simulink model "DraftSimpleEstimatorANDControl"  (R2021b)
settings: Solver=ode1  StartTime=0.0  StopTime=inf  FixedStep=10e-3  RelTol=1e-3
libraries: TcTargetLib x19, slpidlib x1
settings Model: Creator=Mergin  LastModifiedBy=ATLabor
settings OptimizationCC: DefaultParameterBehavior=Inlined  LocalBlockOutputs=off
settings DebuggingCC: UnconnectedInputMsg=none  UnconnectedOutputMsg=none  UnconnectedLineMsg=none
settings ModelReferenceCC: EnableRefExpFcnMdlSchedulingChecks=off
settings RTWCC: Description=TwinCAT GRT Target  SystemTargetFile=TwinCatGrt.tlc  GenCodeOnly=on  TemplateMakefile=tcgrt_msbuild.tmf  TargetLang=C++  DLArmComputeVersion=20.02.1
settings STFCustomTargetCC: TargetLangStandard=C++11 (ISO)  CombineOutputUpdateFcns=on  CodeInterfacePackaging=Reusable function  CPPClassGenCompliant=on  GRTInterface=off  GenerateAllocFcn=on  SystemTargetFile=TwinCatGrt.tlc
settings GRTTargetCC: TargetLangStandard=C++11 (ISO)  ParMdlRefBuildCompliant=off  CompOptLevelCompliant=off  ConcurrentExecutionCompliant=off  MatFileLogging=off  CodeInterfacePackaging=Reusable function  GenerateAllocFcn=on  UseToolchainInfoCompliant=off  ExtModeMexFile=TcExtModeClient

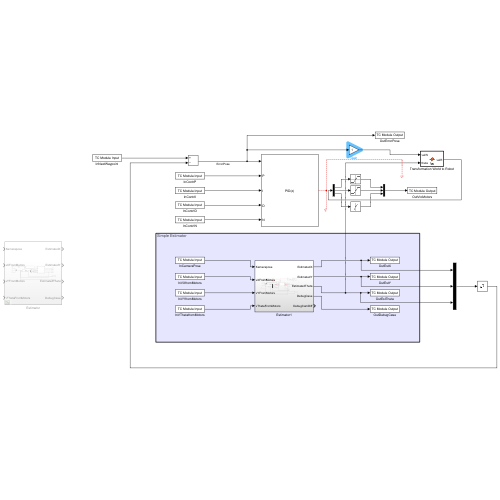
[thumbnail: Simulink's stored preview of the top-level diagram]
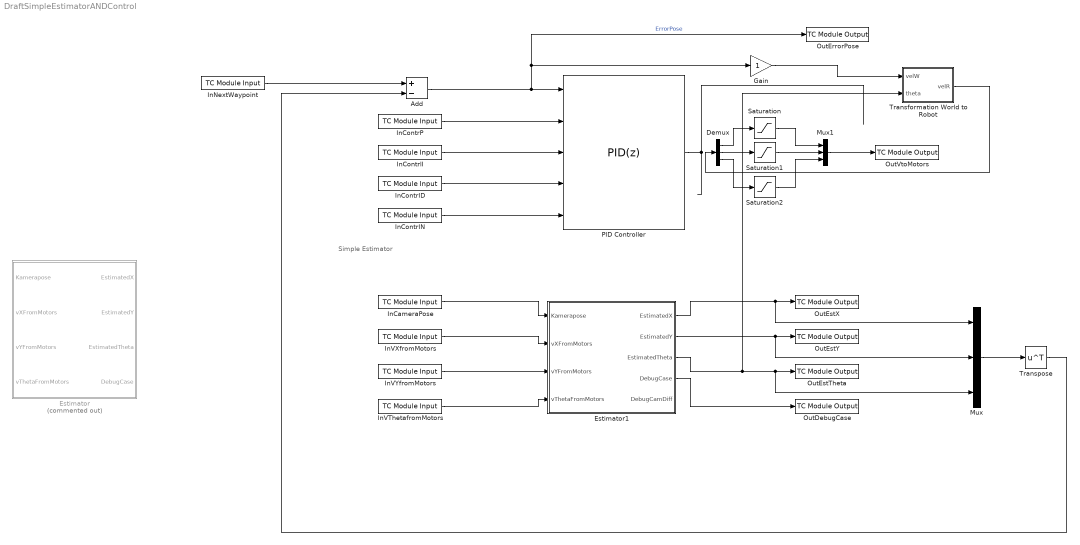
== system DraftSimpleEstimatorANDControl ==
  note: Simple Estimator
  Add : Sum  Inputs=+-
  Demux : Demux  Outputs=3
  Estimator : Subsystem  Commented=on
  Estimator1 : Subsystem
  Gain : Gain
  InCameraPose : TcTargetLib/TC Module Input  PortDataType=double  PortDim=3  Value=[0 0 0]  SampleTime=-1  CodeGenConnectType=DataArea (InputDst)  DataTypeOverride=on
      settings: SourceProductName=Beckhoff TwinCAT Target
  InContrID : TcTargetLib/TC Module Input  PortDataType=double  PortDim=1  Value=0  SampleTime=-1  CodeGenConnectType=DataArea (InputDst)  DataTypeOverride=off
      settings: SourceProductName=Beckhoff TwinCAT Target
  InContrIN : TcTargetLib/TC Module Input  PortDataType=double  PortDim=1  Value=0  SampleTime=-1  CodeGenConnectType=DataArea (InputDst)  DataTypeOverride=off
      settings: SourceProductName=Beckhoff TwinCAT Target
  InContrP : TcTargetLib/TC Module Input  PortDataType=double  PortDim=1  Value=0  SampleTime=-1  CodeGenConnectType=DataArea (InputDst)  DataTypeOverride=off
      settings: SourceProductName=Beckhoff TwinCAT Target
  InContrlI : TcTargetLib/TC Module Input  PortDataType=double  PortDim=1  Value=0  SampleTime=-1  CodeGenConnectType=DataArea (InputDst)  DataTypeOverride=off
      settings: SourceProductName=Beckhoff TwinCAT Target
  InNextWaypoint : TcTargetLib/TC Module Input  PortDataType=double  PortDim=3  Value=[0; 0; 0]  SampleTime=-1  CodeGenConnectType=DataArea (InputDst)  DataTypeOverride=off
      settings: SourceProductName=Beckhoff TwinCAT Target
  InVThetafromMotors : TcTargetLib/TC Module Input  PortDataType=double  PortDim=1  Value=0  SampleTime=-1  CodeGenConnectType=DataArea (InputDst)  DataTypeOverride=off
      settings: SourceProductName=Beckhoff TwinCAT Target
  InVXfromMotors : TcTargetLib/TC Module Input  PortDataType=double  PortDim=1  Value=0  SampleTime=-1  CodeGenConnectType=DataArea (InputDst)  DataTypeOverride=off
      settings: SourceProductName=Beckhoff TwinCAT Target
  InVYfromMotors : TcTargetLib/TC Module Input  PortDataType=double  PortDim=1  Value=0  SampleTime=-1  CodeGenConnectType=DataArea (InputDst)  DataTypeOverride=off
      settings: SourceProductName=Beckhoff TwinCAT Target
  Mux : Mux  Inputs=3
  Mux1 : Mux  Inputs=3
  OutDebugCase : TcTargetLib/TC Module Output  PortDataType=double  PortDim=1  SampleTime=-1  CodeGenConnectType=DataArea (OutputSrc)  DataTypeOverride=off
      settings: SourceProductName=Beckhoff TwinCAT Target
  OutErrorPose : TcTargetLib/TC Module Output  PortDataType=double  PortDim=3  SampleTime=-1  CodeGenConnectType=DataArea (OutputSrc)  DataTypeOverride=off
      settings: SourceProductName=Beckhoff TwinCAT Target
  OutEstTheta : TcTargetLib/TC Module Output  PortDataType=double  PortDim=1  SampleTime=-1  CodeGenConnectType=DataArea (OutputSrc)  DataTypeOverride=off
      settings: SourceProductName=Beckhoff TwinCAT Target
  OutEstX : TcTargetLib/TC Module Output  PortDataType=double  PortDim=1  SampleTime=-1  CodeGenConnectType=DataArea (OutputSrc)  DataTypeOverride=off
      settings: SourceProductName=Beckhoff TwinCAT Target
  OutEstY : TcTargetLib/TC Module Output  PortDataType=double  PortDim=1  SampleTime=-1  CodeGenConnectType=DataArea (OutputSrc)  DataTypeOverride=off
      settings: SourceProductName=Beckhoff TwinCAT Target
  OutVtoMotors : TcTargetLib/TC Module Output  PortDataType=double  PortDim=3  SampleTime=-1  CodeGenConnectType=DataArea (OutputSrc)  DataTypeOverride=off
      settings: SourceProductName=Beckhoff TwinCAT Target
  PID Controller : slpidlib/PID Controller  Controller=PID  Form=Parallel  TimeDomain=Discrete-time  UseExternalTs=off  SampleTime=-1  IntegratorMethod=Forward Euler  FilterMethod=Forward Euler  ControllerParametersSource=external  P=1  I=1  D=0  UseFilter=on  N=100  TunerSelectOption=Transfer Function Based (PID Tuner App)  InitialConditionSource=internal  InitialConditionForIntegrator=0  InitialConditionForFilter=0  DifferentiatorICPrevScaledInput=0  ExternalReset=none  TrackingMode=off  Kt=1  LimitOutput=off  SatLimitsSource=internal  UpperSaturationLimit=inf  LowerSaturationLimit=-inf  LinearizeAsGain=on  AntiWindupMode=none  Kb=1  POutMin=[]  POutMax=[]  IOutMin=[]  IOutMax=[]  DOutMin=[]  DOutMax=[]  NOutMin=[]  NOutMax=[]  SumOutMin=[]  SumOutMax=[]  SaturationOutMin=[]  SaturationOutMax=[]  PParamMin=[]  PParamMax=[]  IParamMin=[]  IParamMax=[]  DParamMin=[]  DParamMax=[]  NParamMin=[]  NParamMax=[]  KbParamMin=[]  KbParamMax=[]  KtParamMin=[]  KtParamMax=[]  KbOutMin=[]  KbOutMax=[]  KtOutMin=[]  KtOutMax=[]  IntegratorOutMin=[]  IntegratorOutMax=[]  FilterOutMin=[]  FilterOutMax=[]  SumI1OutMin=[]  SumI1OutMax=[]  SumI2OutMin=[]  SumI2OutMax=[]  SumI3OutMin=[]  SumI3OutMax=[]  SumI4OutMin=[]  SumI4OutMax=[]  SumDOutMin=[]  SumDOutMax=[]  DifferentiatorOutMin=[]  DifferentiatorOutMax=[]  FilterDiffOutCoefMin=[]  FilterDiffOutCoefMax=[]  ReciprocalOutMin=[]  ReciprocalOutMax=[]  SumDenOutMin=[]  SumDenOutMax=[]  SumNumOutMin=[]  SumNumOutMax=[]  DivideOutMin=[]  DivideOutMax=[]  UdiffTsProdOutMin=[]  UdiffTsProdOutMax=[]  NTsProdOutMin=[]  NTsProdOutMax=[]  UintegralTsProdOutMin=[]  UintegralTsProdOutMax=[]  UngainTsProdOutMin=[]  UngainTsProdOutMax=[]  IntegratorContinuousStateAttributes=''  IntegratorStateMustResolveToSignalObject=off  IntegratorRTWStateStorageClass=Auto  FilterContinuousStateAttributes=''  FilterStateMustResolveToSignalObject=off  FilterRTWStateStorageClass=Auto  ParallelPVariant=ExternalParameters  IdealPVariant=Disabled  IVariant=ExternalParameters  DVariant=ExternalParameters  IntegratorVariant=Discrete  SatVariant=Disabled  AWVariant=Passthrough  PCopyVariant=Disabled  TRVariant=Disabled  FdbkBlocksVariant=Forward  IdealPFdbkVariant=Disabled  SatFdbkVariant=Disabled  DerivativeFilterVariant=ForwardEulerFilter  NVariant=ExternalParameters  NCopyVariant=Disabled  FilterICVariant=InternalICsFilter  IntegratorICVariant=InternalICs  ExternalResetVariant=Disabled  TRSumVariant=Passthrough  SumFdbkVariant=Disabled  SumVariant=Sum_PID  TsampFilterVariant=InternalTs  TsampNgainVariant=Passthrough  TsampIntegralVariant=Passthrough  ExternalSaturationOutDataTypeStr=Inherit: Same as second input
  Saturation : Saturate  UpperLimit=500  LowerLimit=-500
  Saturation1 : Saturate  UpperLimit=500  LowerLimit=-500
  Saturation2 : Saturate  UpperLimit=1  LowerLimit=-1
  Transformation World to Robot : MATLAB Function  TreatAsAtomicUnit=on
  Transpose : Math  Operator=transpose  SaturateOnIntegerOverflow=on
  wires:
  InCameraPose/1 -> Estimator1/1(Kamerapose)
  InVXfromMotors/1 -> Estimator1/2(vXFromMotors)
  InVYfromMotors/1 -> Estimator1/3(vYFromMotors)
  InVThetafromMotors/1 -> Estimator1/4(vThetaFromMotors)
  Estimator1/4(DebugCase) -> OutDebugCase/1
  InContrP/1 -> PID Controller/2
  InContrlI/1 -> PID Controller/3
  InContrID/1 -> PID Controller/4
  InContrIN/1 -> PID Controller/5
  InNextWaypoint/1 -> Add/1
  Add/1 -> Gain/1, OutErrorPose/1, PID Controller/1  "ErrorPose"
  Estimator1/1(EstimatedX) -> OutEstX/1, Mux/1
  Transpose/1 -> Add/2
  Estimator1/2(EstimatedY) -> OutEstY/1, Mux/2
  Mux/1 -> Transpose/1
  Estimator1/3(EstimatedTheta) -> Transformation World to Robot/2(theta), OutEstTheta/1, Mux/3
  PID Controller/1 -> ?
  Demux/1 -> Saturation/1
  Saturation/1 -> Mux1/1
  Demux/2 -> Saturation1/1
  Saturation1/1 -> Mux1/2
  Demux/3 -> Saturation2/1
  Saturation2/1 -> Mux1/3
  Gain/1 -> Transformation World to Robot/1(velW)
  Mux1/1 -> OutVtoMotors/1
  Transformation World to Robot/1(velR) -> Demux/1

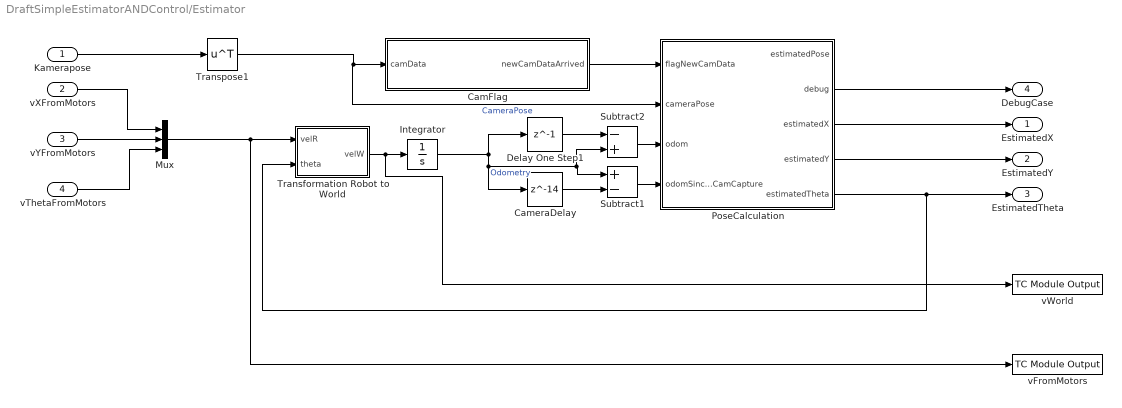
== system DraftSimpleEstimatorANDControl/Estimator ==
  Kamerapose : Inport
  vXFromMotors : Inport  Port=2
  vYFromMotors : Inport  Port=3
  vThetaFromMotors : Inport  Port=4
  CamFlag : MATLAB Function  TreatAsAtomicUnit=on
  CameraDelay : Delay  DelayLength=14
  Delay One Step1 : Delay  DelayLength=1
  Integrator : Integrator
  Mux : Mux  Inputs=3
  PoseCalculation : MATLAB Function  TreatAsAtomicUnit=on
  Subtract1 : Sum  Inputs=+-
  Subtract2 : Sum  Inputs=-+
  Transformation Robot to World : MATLAB Function  TreatAsAtomicUnit=on
  Transpose1 : Math  Operator=transpose  SaturateOnIntegerOverflow=on
  vFromMotors : TcTargetLib/TC Module Output  PortDataType=double  PortDim=3  SampleTime=-1  CodeGenConnectType=DataArea (OutputSrc)  DataTypeOverride=off
      settings: SourceProductName=Beckhoff TwinCAT Target
  vWorld : TcTargetLib/TC Module Output  PortDataType=double  PortDim=3  SampleTime=-1  CodeGenConnectType=DataArea (OutputSrc)  DataTypeOverride=off
      settings: SourceProductName=Beckhoff TwinCAT Target
  EstimatedX : Outport
  EstimatedY : Outport  Port=2
  EstimatedTheta : Outport  Port=3
  DebugCase : Outport  Port=4
  wires:
  vThetaFromMotors/1 -> Mux/3
  Subtract1/1 -> PoseCalculation/4(odomSinceCamCapture)
  CameraDelay/1 -> Subtract1/2
  Transformation Robot to World/1(velW) -> vWorld/1, Integrator/1
  vXFromMotors/1 -> Mux/1
  Transpose1/1 -> CamFlag/1(camData), PoseCalculation/2(cameraPose)  "CameraPose"
  Integrator/1 -> Delay One Step1/1, CameraDelay/1, Subtract2/2, Subtract1/1  "Odometry"
  vYFromMotors/1 -> Mux/2
  CamFlag/1(newCamDataArrived) -> PoseCalculation/1(flagNewCamData)
  Kamerapose/1 -> Transpose1/1
  Delay One Step1/1 -> Subtract2/1
  Subtract2/1 -> PoseCalculation/3(odom)
  PoseCalculation/2(debug) -> DebugCase/1
  Mux/1 -> Transformation Robot to World/1(velR), vFromMotors/1
  PoseCalculation/4(estimatedY) -> EstimatedY/1
  PoseCalculation/3(estimatedX) -> EstimatedX/1
  PoseCalculation/5(estimatedTheta) -> Transformation Robot to World/2(theta), EstimatedTheta/1

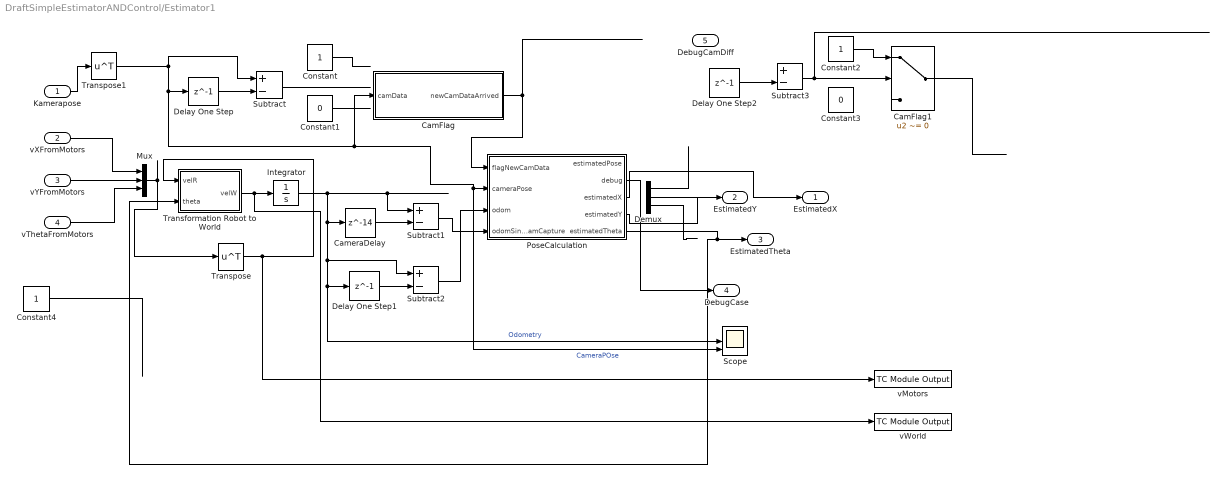
== system DraftSimpleEstimatorANDControl/Estimator1 ==
  Kamerapose : Inport
  vXFromMotors : Inport  Port=2
  vYFromMotors : Inport  Port=3
  vThetaFromMotors : Inport  Port=4
  CamFlag : MATLAB Function  TreatAsAtomicUnit=on
  CamFlag1 : Switch  Criteria=u2 ~= 0
  CameraDelay : Delay  DelayLength=14
  Constant : Constant
  Constant1 : Constant  Value=0
  Constant2 : Constant
  Constant3 : Constant  Value=0
  Constant4 : Constant
  Delay One Step : Delay  DelayLength=1
  Delay One Step1 : Delay  DelayLength=1
  Delay One Step2 : Delay  DelayLength=1
  Demux : Demux  Outputs=3
  Integrator : Integrator
  Mux : Mux  Inputs=3
  PoseCalculation : MATLAB Function  TreatAsAtomicUnit=on
  Scope : Scope  NumInputPorts=3
  Subtract{,1..3} (4 alike) : Sum  Inputs=+-
  Transformation Robot to World : MATLAB Function  TreatAsAtomicUnit=on
  Transpose : Math  Operator=transpose  SaturateOnIntegerOverflow=on
  Transpose1 : Math  Operator=transpose  SaturateOnIntegerOverflow=on
  vMotors : TcTargetLib/TC Module Output  PortDataType=double  PortDim=3  SampleTime=-1  CodeGenConnectType=DataArea (OutputSrc)  DataTypeOverride=off
      settings: SourceProductName=Beckhoff TwinCAT Target
  vWorld : TcTargetLib/TC Module Output  PortDataType=double  PortDim=3  SampleTime=-1  CodeGenConnectType=DataArea (OutputSrc)  DataTypeOverride=off
      settings: SourceProductName=Beckhoff TwinCAT Target
  EstimatedX : Outport
  EstimatedY : Outport  Port=2
  EstimatedTheta : Outport  Port=3
  DebugCase : Outport  Port=4
  DebugCamDiff : Outport  Port=5
  wires:
  Demux/1 -> ?
  Constant/1 -> ?
  Delay One Step/1 -> Subtract/2
  Demux/2 -> ?
  vThetaFromMotors/1 -> Mux/3
  Subtract1/1 -> PoseCalculation/4(odomSinceCamCapture)
  Mux/1 -> Transpose/1
  CameraDelay/1 -> Subtract1/2
  Constant1/1 -> ?
  Transformation Robot to World/1(velW) -> vWorld/1, Integrator/1
  vXFromMotors/1 -> Mux/1
  Transpose1/1 -> Scope/3, PoseCalculation/2(cameraPose), CamFlag/1(camData), Delay One Step/1, Subtract/1  "CameraPOse"
  Integrator/1 -> Subtract1/1, Delay One Step1/1, Scope/2, Subtract2/1, CameraDelay/1  "Odometry"
  vYFromMotors/1 -> Mux/2
  CamFlag/1(newCamDataArrived) -> PoseCalculation/1(flagNewCamData)
  ? -> Scope/1, Demux/1
  Subtract/1 -> ?
  Kamerapose/1 -> Transpose1/1
  Delay One Step1/1 -> Subtract2/2
  Subtract2/1 -> PoseCalculation/3(odom)
  PoseCalculation/2(debug) -> DebugCase/1
  Constant2/1 -> CamFlag1/1
  CamFlag1/1 -> ?
  Subtract3/1 -> CamFlag1/2
  ? -> Subtract3/1  "CameraPOse"
  Delay One Step2/1 -> Subtract3/2
  Transpose/1 -> vMotors/1, Transformation Robot to World/1(velR)
  Demux/3 -> ?
  PoseCalculation/4(estimatedY) -> EstimatedY/1
  PoseCalculation/3(estimatedX) -> EstimatedX/1
  Constant4/1 -> ?
  PoseCalculation/5(estimatedTheta) -> Transformation Robot to World/2(theta), EstimatedTheta/1

== matlab function DraftSimpleEstimatorANDControl/Estimator/PoseCalculation ==
  settings: updateMethod=DISCRETE
  data: flagNewCamData input; cameraPose input; estimatedPose output; odom input; odomSinceCamCapture input; debug output; estimatedX output; estimatedY output; estimatedTheta output
function [estimatedPose, debug, estimatedX, estimatedY, estimatedTheta]= fcn(flagNewCamData, cameraPose, odom, odomSinceCamCapture)

% Variables
persistent estPoseOld

if isempty(estPoseOld)
    estPoseOld = [0 0 0];
end

    % Case 1: Camera Flag is set (New Cameradata) and CameraData is valid
if flagNewCamData == 1
    estimatedPose = cameraPose(1:3) + odomSinceCamCapture;   %OdomSinceCamCapture describes the pose changes since the camera captured the position because the camera data is delayed. in this time the robot drives further.
    estPoseOld = estimatedPose;
    debug = 1;

    % Case 2: No new Cameradata or invalid Cmeradata (integrate transformed velocities of
    % roboter in worldframe
else
    estimatedPose = estPoseOld + odom;
    estPoseOld = estimatedPose;
    debug =2;
end

estimatedX = estimatedPose(1);
estimatedY = estimatedPose(2);
estimatedTheta = estimatedPose(3);

== matlab function DraftSimpleEstimatorANDControl/Estimator/Transformation Robot to World ==
  data: velR input; velW output size=[3 1]; theta input
function velW = fcn(velR, theta)
    TMat = [cos(theta)    -sin(theta)   0;
            sin(theta)    cos(theta)    0;
            0             0             1];
    velW = TMat*velR;
end

== matlab function DraftSimpleEstimatorANDControl/Estimator/CamFlag ==
  data: camData input; newCamDataArrived output
function newCamDataArrived = fcn(camData)

persistent oldCamData

if isempty(oldCamData)
    oldCamData = [0 0 0];
end

if camData ~= oldCamData
    newCamDataArrived = true;
else
    newCamDataArrived = false;
    oldCamData = camData;
end

== matlab function DraftSimpleEstimatorANDControl/Estimator1/CamFlag ==
  data: camData input; newCamDataArrived output
function newCamDataArrived = fcn(camData)

persistent oldCamData

if isempty(oldCamData)
    oldCamData = [0 0 0];
end

if camData ~= oldCamData
    newCamDataArrived = true;
else
    newCamDataArrived = false;
    oldCamData = camData;
end

== matlab function DraftSimpleEstimatorANDControl/Estimator1/PoseCalculation ==
  settings: updateMethod=DISCRETE
  data: flagNewCamData input; cameraPose input; estimatedPose output; odom input; odomSinceCamCapture input; debug output; estimatedX output; estimatedY output; estimatedTheta output
function [estimatedPose, debug, estimatedX, estimatedY, estimatedTheta]= fcn(flagNewCamData, cameraPose, odom, odomSinceCamCapture)

% Variables
persistent estPoseOld

if isempty(estPoseOld)
    estPoseOld = [0 0 0];
end

    % Case 1: Camera Flag is set (New Cameradata) and CameraData is valid
if flagNewCamData == 1
    estimatedPose = cameraPose(1:3) + odomSinceCamCapture;   %OdomSinceCamCapture describes the pose changes since the camera captured the position because the camera data is delayed. in this time the robot drives further.
    estPoseOld = estimatedPose;
    debug = 1;

    % Case 2: No new Cameradata or invalid Cmeradata (integrate transformed velocities of
    % roboter in worldframe
else
    estimatedPose = estPoseOld + odom;
    estPoseOld = estimatedPose;
    debug =2;
end

estimatedX = estimatedPose(1);
estimatedY = estimatedPose(2);
estimatedTheta = estimatedPose(3);

== matlab function DraftSimpleEstimatorANDControl/Estimator1/Transformation Robot to World ==
  data: velR input; velW output size=[1 3]; theta input
function velW = fcn(velR, theta)
    TMat = [cos(theta)    -sin(theta)   0;
            sin(theta)    cos(theta)    0;
            0             0             1];
    velW = velR*transpose(TMat);
end

== matlab function DraftSimpleEstimatorANDControl/Transformation World to Robot ==
  data: velW input; velR output size=[3 1]; theta input
function velR = fcn(velW, theta)
    TMat = [cos(theta)     sin(theta)    0;
            -sin(theta)    cos(theta)    0;
            0              0             1];
    velR = TMat*velW;
end
